simulink model "switch_regulator"  (R2019b)
settings: Solver=VariableStepAuto  StartTime=0.0  StopTime=3  RelTol=1e-3
undefined symbols (not defined in the file): J, km, L, R
settings Model: Creator=Gudini  LastModifiedBy=Gudini

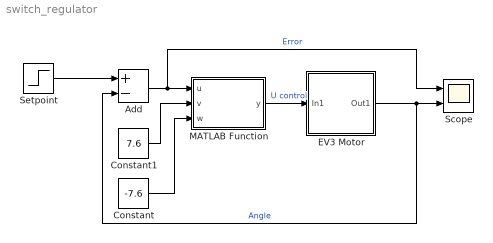
== system switch_regulator ==
  Add : Sum  Inputs=+-
  Constant : Constant  Value=-7.6
  Constant1 : Constant  Value=7.6
  EV3 Motor : Subsystem
  MATLAB Function : MATLAB Function  TreatAsAtomicUnit=on
  Scope : Scope  NumInputPorts=2
  "Setpoint " : Step  After=3.14  SampleTime=0
  wires:
  Add/1 -> Scope/1, MATLAB Function/1(u)  "Error"
  "Setpoint "/1 -> Add/1
  EV3 Motor/1(Out1) -> Add/2, Scope/2  "Angle"
  Constant1/1 -> MATLAB Function/2(v)
  Constant/1 -> MATLAB Function/3(w)
  MATLAB Function/1(y) -> EV3 Motor/1(In1)  "U control"

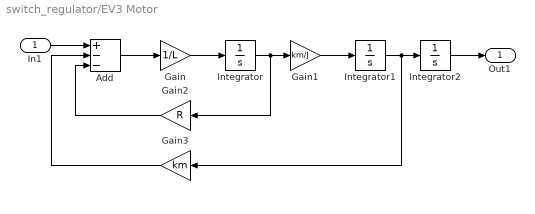
== system switch_regulator/EV3 Motor ==
  In1 : Inport
  Add : Sum  Inputs=+--
  Gain : Gain  Gain=1/L
  Gain1 : Gain  Gain=km/J
  Gain2 : Gain  Gain=R
  Gain3 : Gain  Gain=km
  Integrator : Integrator
  Integrator1 : Integrator
  Integrator2 : Integrator
  Out1 : Outport
  wires:
  Gain1/1 -> Integrator1/1
  Integrator1/1 -> Gain3/1, Integrator2/1
  In1/1 -> Add/1
  Integrator2/1 -> Out1/1
  Integrator/1 -> Gain2/1, Gain1/1
  Gain/1 -> Integrator/1
  Gain2/1 -> Add/3
  Add/1 -> Gain/1
  Gain3/1 -> Add/2

== matlab function switch_regulator/MATLAB Function ==
  data: u input; y output; v input; w input
function y = fcn(u, v, w)
if u == 0
   y = 0;
elseif u > 0
   y = v;
else
   y = w;
end
